simulink model "RightReachDemo"  (Simulink 6.2)
settings: Solver=ode45  StartTime=0.0  StopTime=10.0  RelTol=1e-3
settings Model: LastModifiedBy=suarezjl
settings DataIOCC: SignalLoggingName=sigsOut
settings HardwareCC: TargetUnknown=on

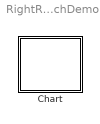
== system RightReachDemo ==
  Chart : Stateflow chart

== stateflow chart Chart ==
  state StartCameras
    \\Popeye\RightReachDemo\RightArm\StateMachine.LoadSM()
    \\Popeye\RightReachDemo\RightArm\StateMachine.Start()
    \\Popeye\RightReachDemo\RightTrajectoryAgent\StateMachine.LoadSM()
    \\Popeye\RightReachDemo\RightTrajectoryAgent\StateMachine.Start()
  state Stop
    \\Popeye\RightReachDemo\RightArm\StateMachine.Stop()
    \\Popeye\RightReachDemo\RightTrajectoryAgent\StateMachine.Stop()
  (default) -> StartCameras : Start
  StartCameras -> Stop : Signal="Stop"
